simulink model "FSAC2021"  (R2014a)
settings: Solver=FixedStepDiscrete  StartTime=0.0  StopTime=inf  FixedStep=0.0005  RelTol=1e-3
model workspace (MAT data in the model file):
  MCOS : class17 (value not decoded)
  MCOS : class17 (value not decoded)
  MCOS : class17 (value not decoded)
  MCOS : class17 (value not decoded)
  MCOS : class17 (value not decoded)
  MCOS : class17 (value not decoded)
  MCOS : class17 (value not decoded)
  MCOS : class17 (value not decoded)
  MCOS : class17 (value not decoded)
  MCOS : class17 (value not decoded)
  MCOS : class17 (value not decoded)
  MCOS : class17 (value not decoded)
  MCOS : class17 (value not decoded)
  MCOS : class17 (value not decoded)
  MCOS : class17 (value not decoded)
  MCOS : class17 (value not decoded)
  MCOS : class17 (value not decoded)
  MCOS : class17 (value not decoded)
  MCOS : class17 (value not decoded)
  BUZZER_START = 1
  MCOS : class17 (value not decoded)
  MCOS : class17 (value not decoded)
  MCOS : class17 (value not decoded)
  MCOS : class17 (value not decoded)
  MCOS : class17 (value not decoded)
  MCOS : class17 (value not decoded)
  MCOS : class17 (value not decoded)
  MCOS : class17 (value not decoded)
  MCOS : class17 (value not decoded)
  MCOS : class17 (value not decoded)
  MCOS : class17 (value not decoded)
  MCOS : class17 (value not decoded)
  MCOS : class17 (value not decoded)
  MCOS : class17 (value not decoded)
  MCOS : class17 (value not decoded)
  MCOS : class17 (value not decoded)
  MCOS : class17 (value not decoded)
  MCOS : class17 (value not decoded)
  MCOS : class17 (value not decoded)
  MCOS : class17 (value not decoded)
  MCOS : class17 (value not decoded)
  MCOS : class17 (value not decoded)
  MCOS : class17 (value not decoded)
  MCOS : class17 (value not decoded)
  MCOS : class17 (value not decoded)
  MCOS : class17 (value not decoded)
  MCOS : class17 (value not decoded)
  MCOS : class17 (value not decoded)
  MCOS : class17 (value not decoded)
  MCOS : class17 (value not decoded)
  MCOS : class17 (value not decoded)
  MCOS : class17 (value not decoded)
  MCOS : class17 (value not decoded)
  MCOS : class17 (value not decoded)
  MCOS : class17 (value not decoded)
  MCOS : class17 (value not decoded)
  MCOS : class17 (value not decoded)
  MCOS : class17 (value not decoded)
  Brake = 11
  MCOS : class17 (value not decoded)
  MCOS : class17 (value not decoded)
  MCOS : class17 (value not decoded)
  MCOS : class17 (value not decoded)
  MCOS : class17 (value not decoded)
  MCOS : class17 (value not decoded)
  MCOS : class17 (value not decoded)
  MCOS : class17 (value not decoded)
  Sensor_Acc_b = 101.85
  Sensor_Acc_k = -0.0185
  Str_Sen_Orig_Angle = -341
  MCOS : class17 (value not decoded)
  Tire_D = 0.47
  T = 0.05
libraries: simulink x396, ec55xxlib x126
(part 10 of 17)

== system FSAC2021/ROUTING/TO_DCAN/Subsystem/DIAG_VEH_INFO ==
  Volt_Cmp_Mtr_Sts_in : Inport
  Volt_Cmp_BMS_Sts_in : Inport  Port=2
  Hydra_Prs_SN_Sts_in : Inport  Port=3
  EBS_Gas_SN_2_Sts_in : Inport  Port=4
  EBS_Gas_SN_1_Sts_in : Inport  Port=5
  Brk_Disp_SN_Sts_in : Inport  Port=6
  Acc_SN_2_Sts_in : Inport  Port=7
  Acc_SN_1_Sts_in : Inport  Port=8
  Point_VCU_in : Inport  Port=9
  Point_StrSr_in : Inport  Port=10
  Point_SCU_in : Inport  Port=11
  Point_RES_in : Inport  Port=12
  Point_MCU_in : Inport  Port=13
  Point_IPC_in : Inport  Port=14
  Point_Drive_Motor_in : Inport  Port=15
  Point_BMS_in : Inport  Port=16
  Point_BCU_in : Inport  Port=17
  Start_Swtich_in : Inport  Port=18
  On_Out_Switch_in : Inport  Port=19
  On_In_Swtich_in : Inport  Port=20
  LV_Switch_in : Inport  Port=21
  HV_Switch_in : Inport  Port=22
  EBS_Rls_Switch_in : Inport  Port=23
  ASMS_Swtich_in : Inport  Port=24
  AMI_State_in : Inport  Port=25
  High_voltage_on_in : Inport  Port=26
  EBS_Status_in : Inport  Port=27
  EBS_Fault_in : Inport  Port=28
  AS_State_in : Inport  Port=29
  AMI_State : Subsystem
  ASMS_Swtich : Subsystem
  AS_State : Subsystem
  Acc_SN_1_Sts : Subsystem
  Acc_SN_2_Sts : Subsystem
  Brk_Disp_SN_Sts : Subsystem
  Conv{1..8} (8 alike) : DataTypeConversion
  DIAG_VEH_INFO_DLC : Constant  Value=8  OutDataTypeStr=uint8
  DIAG_VEH_INFO_DLC_Out : Terminator
  DIAG_VEH_INFO_ID : Constant  Value=1905  OutDataTypeStr=single
  DIAG_VEH_INFO_ID_Out : Terminator
  DIAG_VEH_INFO_mux : Mux  Inputs=8
  EBS_Fault : Subsystem
  EBS_Gas_SN_1_Sts : Subsystem
  EBS_Gas_SN_2_Sts : Subsystem
  EBS_Rls_Switch : Subsystem
  EBS_Status : Subsystem
  HV_Switch : Subsystem
  High_voltage_on : Subsystem
  Hydra_Prs_SN_Sts : Subsystem
  LV_Switch : Subsystem
  On_In_Swtich : Subsystem
  On_Out_Switch : Subsystem
  Point_BCU : Subsystem
  Point_BMS : Subsystem
  Point_Drive_Motor : Subsystem
  Point_IPC : Subsystem
  Point_MCU : Subsystem
  Point_RES : Subsystem
  Point_SCU : Subsystem
  Point_StrSr : Subsystem
  Point_VCU : Subsystem
  Start_Swtich : Subsystem
  Volt_Cmp_BMS_Sts : Subsystem
  Volt_Cmp_Mtr_Sts : Subsystem
  or{1..8} (8 alike) : simulink/Logic and Bit Operations/Bitwise Operator  logicop=OR  UseBitMask=off  NumInputPorts=29  BitMask=bin2dec('11011001')  BitMaskRealWorld=Stored Integer
  output : Outport
  wires:
  DIAG_VEH_INFO_mux/1 -> output/1
  Volt_Cmp_Mtr_Sts/1(output1) -> or1/1
  Volt_Cmp_Mtr_Sts/2(output2) -> or2/1
  Volt_Cmp_Mtr_Sts/3(output3) -> or3/1
  Volt_Cmp_Mtr_Sts/4(output4) -> or4/1
  Volt_Cmp_Mtr_Sts/5(output5) -> or5/1
  Volt_Cmp_Mtr_Sts/6(output6) -> or6/1
  Volt_Cmp_Mtr_Sts/7(output7) -> or7/1
  Volt_Cmp_Mtr_Sts/8(output8) -> or8/1
  Volt_Cmp_BMS_Sts/1(output1) -> or1/2
  Volt_Cmp_BMS_Sts/2(output2) -> or2/2
  Volt_Cmp_BMS_Sts/3(output3) -> or3/2
  Volt_Cmp_BMS_Sts/4(output4) -> or4/2
  Volt_Cmp_BMS_Sts/5(output5) -> or5/2
  Volt_Cmp_BMS_Sts/6(output6) -> or6/2
  Volt_Cmp_BMS_Sts/7(output7) -> or7/2
  Volt_Cmp_BMS_Sts/8(output8) -> or8/2
  Hydra_Prs_SN_Sts/1(output1) -> or1/3
  Hydra_Prs_SN_Sts/2(output2) -> or2/3
  Hydra_Prs_SN_Sts/3(output3) -> or3/3
  Hydra_Prs_SN_Sts/4(output4) -> or4/3
  Hydra_Prs_SN_Sts/5(output5) -> or5/3
  Hydra_Prs_SN_Sts/6(output6) -> or6/3
  Hydra_Prs_SN_Sts/7(output7) -> or7/3
  Hydra_Prs_SN_Sts/8(output8) -> or8/3
  EBS_Gas_SN_2_Sts/1(output1) -> or1/4
  EBS_Gas_SN_2_Sts/2(output2) -> or2/4
  EBS_Gas_SN_2_Sts/3(output3) -> or3/4
  EBS_Gas_SN_2_Sts/4(output4) -> or4/4
  EBS_Gas_SN_2_Sts/5(output5) -> or5/4
  EBS_Gas_SN_2_Sts/6(output6) -> or6/4
  EBS_Gas_SN_2_Sts/7(output7) -> or7/4
  EBS_Gas_SN_2_Sts/8(output8) -> or8/4
  EBS_Gas_SN_1_Sts/1(output1) -> or1/5
  EBS_Gas_SN_1_Sts/2(output2) -> or2/5
  EBS_Gas_SN_1_Sts/3(output3) -> or3/5
  EBS_Gas_SN_1_Sts/4(output4) -> or4/5
  EBS_Gas_SN_1_Sts/5(output5) -> or5/5
  EBS_Gas_SN_1_Sts/6(output6) -> or6/5
  EBS_Gas_SN_1_Sts/7(output7) -> or7/5
  EBS_Gas_SN_1_Sts/8(output8) -> or8/5
  Brk_Disp_SN_Sts/1(output1) -> or1/6
  Brk_Disp_SN_Sts/2(output2) -> or2/6
  Brk_Disp_SN_Sts/3(output3) -> or3/6
  Brk_Disp_SN_Sts/4(output4) -> or4/6
  Brk_Disp_SN_Sts/5(output5) -> or5/6
  Brk_Disp_SN_Sts/6(output6) -> or6/6
  Brk_Disp_SN_Sts/7(output7) -> or7/6
  Brk_Disp_SN_Sts/8(output8) -> or8/6
  Acc_SN_2_Sts/1(output1) -> or1/7
  Acc_SN_2_Sts/2(output2) -> or2/7
  Acc_SN_2_Sts/3(output3) -> or3/7
  Acc_SN_2_Sts/4(output4) -> or4/7
  Acc_SN_2_Sts/5(output5) -> or5/7
  Acc_SN_2_Sts/6(output6) -> or6/7
  Acc_SN_2_Sts/7(output7) -> or7/7
  Acc_SN_2_Sts/8(output8) -> or8/7
  Acc_SN_1_Sts/1(output1) -> or1/8
  Acc_SN_1_Sts/2(output2) -> or2/8
  Acc_SN_1_Sts/3(output3) -> or3/8
  Acc_SN_1_Sts/4(output4) -> or4/8
  Acc_SN_1_Sts/5(output5) -> or5/8
  Acc_SN_1_Sts/6(output6) -> or6/8
  Acc_SN_1_Sts/7(output7) -> or7/8
  Acc_SN_1_Sts/8(output8) -> or8/8
  Point_VCU/1(output1) -> or1/9
  Point_VCU/2(output2) -> or2/9
  Point_VCU/3(output3) -> or3/9
  Point_VCU/4(output4) -> or4/9
  Point_VCU/5(output5) -> or5/9
  Point_VCU/6(output6) -> or6/9
  Point_VCU/7(output7) -> or7/9
  Point_VCU/8(output8) -> or8/9
  Point_StrSr/1(output1) -> or1/10
  Point_StrSr/2(output2) -> or2/10
  Point_StrSr/3(output3) -> or3/10
  Point_StrSr/4(output4) -> or4/10
  Point_StrSr/5(output5) -> or5/10
  Point_StrSr/6(output6) -> or6/10
  Point_StrSr/7(output7) -> or7/10
  Point_StrSr/8(output8) -> or8/10
  Point_SCU/1(output1) -> or1/11
  Point_SCU/2(output2) -> or2/11
  Point_SCU/3(output3) -> or3/11
  Point_SCU/4(output4) -> or4/11
  Point_SCU/5(output5) -> or5/11
  Point_SCU/6(output6) -> or6/11
  Point_SCU/7(output7) -> or7/11
  Point_SCU/8(output8) -> or8/11
  Point_RES/1(output1) -> or1/12
  Point_RES/2(output2) -> or2/12
  Point_RES/3(output3) -> or3/12
  Point_RES/4(output4) -> or4/12
  Point_RES/5(output5) -> or5/12
  Point_RES/6(output6) -> or6/12
  Point_RES/7(output7) -> or7/12
  Point_RES/8(output8) -> or8/12
  Point_MCU/1(output1) -> or1/13
  Point_MCU/2(output2) -> or2/13
  Point_MCU/3(output3) -> or3/13
  Point_MCU/4(output4) -> or4/13
  Point_MCU/5(output5) -> or5/13
  Point_MCU/6(output6) -> or6/13
  Point_MCU/7(output7) -> or7/13
  Point_MCU/8(output8) -> or8/13
  Point_IPC/1(output1) -> or1/14
  Point_IPC/2(output2) -> or2/14
  Point_IPC/3(output3) -> or3/14
  Point_IPC/4(output4) -> or4/14
  Point_IPC/5(output5) -> or5/14
  Point_IPC/6(output6) -> or6/14
  Point_IPC/7(output7) -> or7/14
  Point_IPC/8(output8) -> or8/14
  Point_Drive_Motor/1(output1) -> or1/15
  Point_Drive_Motor/2(output2) -> or2/15
  Point_Drive_Motor/3(output3) -> or3/15
  Point_Drive_Motor/4(output4) -> or4/15
  Point_Drive_Motor/5(output5) -> or5/15
  Point_Drive_Motor/6(output6) -> or6/15
  Point_Drive_Motor/7(output7) -> or7/15
  Point_Drive_Motor/8(output8) -> or8/15
  Point_BMS/1(output1) -> or1/16
  Point_BMS/2(output2) -> or2/16
  Point_BMS/3(output3) -> or3/16
  Point_BMS/4(output4) -> or4/16
  Point_BMS/5(output5) -> or5/16
  Point_BMS/6(output6) -> or6/16
  Point_BMS/7(output7) -> or7/16
  Point_BMS/8(output8) -> or8/16
  Point_BCU/1(output1) -> or1/17
  Point_BCU/2(output2) -> or2/17
  Point_BCU/3(output3) -> or3/17
  Point_BCU/4(output4) -> or4/17
  Point_BCU/5(output5) -> or5/17
  Point_BCU/6(output6) -> or6/17
  Point_BCU/7(output7) -> or7/17
  Point_BCU/8(output8) -> or8/17
  Start_Swtich/1(output1) -> or1/18
  Start_Swtich/2(output2) -> or2/18
  Start_Swtich/3(output3) -> or3/18
  Start_Swtich/4(output4) -> or4/18
  Start_Swtich/5(output5) -> or5/18
  Start_Swtich/6(output6) -> or6/18
  Start_Swtich/7(output7) -> or7/18
  Start_Swtich/8(output8) -> or8/18
  On_Out_Switch/1(output1) -> or1/19
  On_Out_Switch/2(output2) -> or2/19
  On_Out_Switch/3(output3) -> or3/19
  On_Out_Switch/4(output4) -> or4/19
  On_Out_Switch/5(output5) -> or5/19
  On_Out_Switch/6(output6) -> or6/19
  On_Out_Switch/7(output7) -> or7/19
  On_Out_Switch/8(output8) -> or8/19
  On_In_Swtich/1(output1) -> or1/20
  On_In_Swtich/2(output2) -> or2/20
  On_In_Swtich/3(output3) -> or3/20
  On_In_Swtich/4(output4) -> or4/20
  On_In_Swtich/5(output5) -> or5/20
  On_In_Swtich/6(output6) -> or6/20
  On_In_Swtich/7(output7) -> or7/20
  On_In_Swtich/8(output8) -> or8/20
  LV_Switch/1(output1) -> or1/21
  LV_Switch/2(output2) -> or2/21
  LV_Switch/3(output3) -> or3/21
  LV_Switch/4(output4) -> or4/21
  LV_Switch/5(output5) -> or5/21
  LV_Switch/6(output6) -> or6/21
  LV_Switch/7(output7) -> or7/21
  LV_Switch/8(output8) -> or8/21
  HV_Switch/1(output1) -> or1/22
  HV_Switch/2(output2) -> or2/22
  HV_Switch/3(output3) -> or3/22
  HV_Switch/4(output4) -> or4/22
  HV_Switch/5(output5) -> or5/22
  HV_Switch/6(output6) -> or6/22
  HV_Switch/7(output7) -> or7/22
  HV_Switch/8(output8) -> or8/22
  EBS_Rls_Switch/1(output1) -> or1/23
  EBS_Rls_Switch/2(output2) -> or2/23
  EBS_Rls_Switch/3(output3) -> or3/23
  EBS_Rls_Switch/4(output4) -> or4/23
  EBS_Rls_Switch/5(output5) -> or5/23
  EBS_Rls_Switch/6(output6) -> or6/23
  EBS_Rls_Switch/7(output7) -> or7/23
  EBS_Rls_Switch/8(output8) -> or8/23
  ASMS_Swtich/1(output1) -> or1/24
  ASMS_Swtich/2(output2) -> or2/24
  ASMS_Swtich/3(output3) -> or3/24
  ASMS_Swtich/4(output4) -> or4/24
  ASMS_Swtich/5(output5) -> or5/24
  ASMS_Swtich/6(output6) -> or6/24
  ASMS_Swtich/7(output7) -> or7/24
  ASMS_Swtich/8(output8) -> or8/24
  AMI_State/1(output1) -> or1/25
  AMI_State/2(output2) -> or2/25
  AMI_State/3(output3) -> or3/25
  AMI_State/4(output4) -> or4/25
  AMI_State/5(output5) -> or5/25
  AMI_State/6(output6) -> or6/25
  AMI_State/7(output7) -> or7/25
  AMI_State/8(output8) -> or8/25
  High_voltage_on/1(output1) -> or1/26
  High_voltage_on/2(output2) -> or2/26
  High_voltage_on/3(output3) -> or3/26
  High_voltage_on/4(output4) -> or4/26
  High_voltage_on/5(output5) -> or5/26
  High_voltage_on/6(output6) -> or6/26
  High_voltage_on/7(output7) -> or7/26
  High_voltage_on/8(output8) -> or8/26
  EBS_Status/1(output1) -> or1/27
  EBS_Status/2(output2) -> or2/27
  EBS_Status/3(output3) -> or3/27
  EBS_Status/4(output4) -> or4/27
  EBS_Status/5(output5) -> or5/27
  EBS_Status/6(output6) -> or6/27
  EBS_Status/7(output7) -> or7/27
  EBS_Status/8(output8) -> or8/27
  EBS_Fault/1(output1) -> or1/28
  EBS_Fault/2(output2) -> or2/28
  EBS_Fault/3(output3) -> or3/28
  EBS_Fault/4(output4) -> or4/28
  EBS_Fault/5(output5) -> or5/28
  EBS_Fault/6(output6) -> or6/28
  EBS_Fault/7(output7) -> or7/28
  EBS_Fault/8(output8) -> or8/28
  AS_State/1(output1) -> or1/29
  AS_State/2(output2) -> or2/29
  AS_State/3(output3) -> or3/29
  AS_State/4(output4) -> or4/29
  AS_State/5(output5) -> or5/29
  AS_State/6(output6) -> or6/29
  AS_State/7(output7) -> or7/29
  AS_State/8(output8) -> or8/29
  or1/1 -> Conv1/1
  Conv1/1 -> DIAG_VEH_INFO_mux/1
  or2/1 -> Conv2/1
  Conv2/1 -> DIAG_VEH_INFO_mux/2
  or3/1 -> Conv3/1
  Conv3/1 -> DIAG_VEH_INFO_mux/3
  or4/1 -> Conv4/1
  Conv4/1 -> DIAG_VEH_INFO_mux/4
  or5/1 -> Conv5/1
  Conv5/1 -> DIAG_VEH_INFO_mux/5
  or6/1 -> Conv6/1
  Conv6/1 -> DIAG_VEH_INFO_mux/6
  or7/1 -> Conv7/1
  Conv7/1 -> DIAG_VEH_INFO_mux/7
  or8/1 -> Conv8/1
  Conv8/1 -> DIAG_VEH_INFO_mux/8
  DIAG_VEH_INFO_ID/1 -> DIAG_VEH_INFO_ID_Out/1
  DIAG_VEH_INFO_DLC/1 -> DIAG_VEH_INFO_DLC_Out/1
  Volt_Cmp_Mtr_Sts_in/1 -> Volt_Cmp_Mtr_Sts/1(Volt_Cmp_Mtr_Sts)
  Volt_Cmp_BMS_Sts_in/1 -> Volt_Cmp_BMS_Sts/1(Volt_Cmp_BMS_Sts)
  Hydra_Prs_SN_Sts_in/1 -> Hydra_Prs_SN_Sts/1(Hydra_Prs_SN_Sts)
  EBS_Gas_SN_2_Sts_in/1 -> EBS_Gas_SN_2_Sts/1(EBS_Gas_SN_2_Sts)
  EBS_Gas_SN_1_Sts_in/1 -> EBS_Gas_SN_1_Sts/1(EBS_Gas_SN_1_Sts)
  Brk_Disp_SN_Sts_in/1 -> Brk_Disp_SN_Sts/1(Brk_Disp_SN_Sts)
  Acc_SN_2_Sts_in/1 -> Acc_SN_2_Sts/1(Acc_SN_2_Sts)
  Acc_SN_1_Sts_in/1 -> Acc_SN_1_Sts/1(Acc_SN_1_Sts)
  Point_VCU_in/1 -> Point_VCU/1(Point_VCU)
  Point_StrSr_in/1 -> Point_StrSr/1(Point_StrSr)
  Point_SCU_in/1 -> Point_SCU/1(Point_SCU)
  Point_RES_in/1 -> Point_RES/1(Point_RES)
  Point_MCU_in/1 -> Point_MCU/1(Point_MCU)
  Point_IPC_in/1 -> Point_IPC/1(Point_IPC)
  Point_Drive_Motor_in/1 -> Point_Drive_Motor/1(Point_Drive_Motor)
  Point_BMS_in/1 -> Point_BMS/1(Point_BMS)
  Point_BCU_in/1 -> Point_BCU/1(Point_BCU)
  Start_Swtich_in/1 -> Start_Swtich/1(Start_Swtich)
  On_Out_Switch_in/1 -> On_Out_Switch/1(On_Out_Switch)
  On_In_Swtich_in/1 -> On_In_Swtich/1(On_In_Swtich)
  LV_Switch_in/1 -> LV_Switch/1(LV_Switch)
  HV_Switch_in/1 -> HV_Switch/1(HV_Switch)
  EBS_Rls_Switch_in/1 -> EBS_Rls_Switch/1(EBS_Rls_Switch)
  ASMS_Swtich_in/1 -> ASMS_Swtich/1(ASMS_Swtich)
  AMI_State_in/1 -> AMI_State/1(AMI_State)
  High_voltage_on_in/1 -> High_voltage_on/1(High_voltage_on)
  EBS_Status_in/1 -> EBS_Status/1(EBS_Status)
  EBS_Fault_in/1 -> EBS_Fault/1(EBS_Fault)
  AS_State_in/1 -> AS_State/1(AS_State)

== system FSAC2021/ROUTING/TO_DCAN/Subsystem/DIAG_VEH_SENSOR ==
  Pedal_Brake_in : Inport
  Pedal_Acc_in : Inport  Port=2
  Veh_Current_Speed_in : Inport  Port=3
  Front_wheel_angle_in : Inport  Port=4
  Mtr_Input_Volt_in : Inport  Port=5
  BMS_Output_Volt_in : Inport  Port=6
  Hydra_Prs_in : Inport  Port=7
  EBS_Gas_Prs_2_in : Inport  Port=8
  EBS_Gas_Prs_1_in : Inport  Port=9
  BMS_Output_Volt : Subsystem
  Conv{1..8} (8 alike) : DataTypeConversion
  DIAG_VEH_SENSOR_DLC : Constant  Value=8  OutDataTypeStr=uint8
  DIAG_VEH_SENSOR_DLC_Out : Terminator
  DIAG_VEH_SENSOR_ID : Constant  Value=1873  OutDataTypeStr=single
  DIAG_VEH_SENSOR_ID_Out : Terminator
  DIAG_VEH_SENSOR_mux : Mux  Inputs=8
  EBS_Gas_Prs_1 : Subsystem
  EBS_Gas_Prs_2 : Subsystem
  Front_wheel_angle : Subsystem
  Hydra_Prs : Subsystem
  Mtr_Input_Volt : Subsystem
  Pedal_Acc : Subsystem
  Pedal_Brake : Subsystem
  Veh_Current_Speed : Subsystem
  or{1..8} (8 alike) : simulink/Logic and Bit Operations/Bitwise Operator  logicop=OR  UseBitMask=off  NumInputPorts=9  BitMask=bin2dec('11011001')  BitMaskRealWorld=Stored Integer
  output : Outport
  wires:
  DIAG_VEH_SENSOR_mux/1 -> output/1
  Pedal_Brake/1(output1) -> or1/1
  Pedal_Brake/2(output2) -> or2/1
  Pedal_Brake/3(output3) -> or3/1
  Pedal_Brake/4(output4) -> or4/1
  Pedal_Brake/5(output5) -> or5/1
  Pedal_Brake/6(output6) -> or6/1
  Pedal_Brake/7(output7) -> or7/1
  Pedal_Brake/8(output8) -> or8/1
  Pedal_Acc/1(output1) -> or1/2
  Pedal_Acc/2(output2) -> or2/2
  Pedal_Acc/3(output3) -> or3/2
  Pedal_Acc/4(output4) -> or4/2
  Pedal_Acc/5(output5) -> or5/2
  Pedal_Acc/6(output6) -> or6/2
  Pedal_Acc/7(output7) -> or7/2
  Pedal_Acc/8(output8) -> or8/2
  Veh_Current_Speed/1(output1) -> or1/3
  Veh_Current_Speed/2(output2) -> or2/3
  Veh_Current_Speed/3(output3) -> or3/3
  Veh_Current_Speed/4(output4) -> or4/3
  Veh_Current_Speed/5(output5) -> or5/3
  Veh_Current_Speed/6(output6) -> or6/3
  Veh_Current_Speed/7(output7) -> or7/3
  Veh_Current_Speed/8(output8) -> or8/3
  Front_wheel_angle/1(output1) -> or1/4
  Front_wheel_angle/2(output2) -> or2/4
  Front_wheel_angle/3(output3) -> or3/4
  Front_wheel_angle/4(output4) -> or4/4
  Front_wheel_angle/5(output5) -> or5/4
  Front_wheel_angle/6(output6) -> or6/4
  Front_wheel_angle/7(output7) -> or7/4
  Front_wheel_angle/8(output8) -> or8/4
  Mtr_Input_Volt/1(output1) -> or1/5
  Mtr_Input_Volt/2(output2) -> or2/5
  Mtr_Input_Volt/3(output3) -> or3/5
  Mtr_Input_Volt/4(output4) -> or4/5
  Mtr_Input_Volt/5(output5) -> or5/5
  Mtr_Input_Volt/6(output6) -> or6/5
  Mtr_Input_Volt/7(output7) -> or7/5
  Mtr_Input_Volt/8(output8) -> or8/5
  BMS_Output_Volt/1(output1) -> or1/6
  BMS_Output_Volt/2(output2) -> or2/6
  BMS_Output_Volt/3(output3) -> or3/6
  BMS_Output_Volt/4(output4) -> or4/6
  BMS_Output_Volt/5(output5) -> or5/6
  BMS_Output_Volt/6(output6) -> or6/6
  BMS_Output_Volt/7(output7) -> or7/6
  BMS_Output_Volt/8(output8) -> or8/6
  Hydra_Prs/1(output1) -> or1/7
  Hydra_Prs/2(output2) -> or2/7
  Hydra_Prs/3(output3) -> or3/7
  Hydra_Prs/4(output4) -> or4/7
  Hydra_Prs/5(output5) -> or5/7
  Hydra_Prs/6(output6) -> or6/7
  Hydra_Prs/7(output7) -> or7/7
  Hydra_Prs/8(output8) -> or8/7
  EBS_Gas_Prs_2/1(output1) -> or1/8
  EBS_Gas_Prs_2/2(output2) -> or2/8
  EBS_Gas_Prs_2/3(output3) -> or3/8
  EBS_Gas_Prs_2/4(output4) -> or4/8
  EBS_Gas_Prs_2/5(output5) -> or5/8
  EBS_Gas_Prs_2/6(output6) -> or6/8
  EBS_Gas_Prs_2/7(output7) -> or7/8
  EBS_Gas_Prs_2/8(output8) -> or8/8
  EBS_Gas_Prs_1/1(output1) -> or1/9
  EBS_Gas_Prs_1/2(output2) -> or2/9
  EBS_Gas_Prs_1/3(output3) -> or3/9
  EBS_Gas_Prs_1/4(output4) -> or4/9
  EBS_Gas_Prs_1/5(output5) -> or5/9
  EBS_Gas_Prs_1/6(output6) -> or6/9
  EBS_Gas_Prs_1/7(output7) -> or7/9
  EBS_Gas_Prs_1/8(output8) -> or8/9
  or1/1 -> Conv1/1
  Conv1/1 -> DIAG_VEH_SENSOR_mux/1
  or2/1 -> Conv2/1
  Conv2/1 -> DIAG_VEH_SENSOR_mux/2
  or3/1 -> Conv3/1
  Conv3/1 -> DIAG_VEH_SENSOR_mux/3
  or4/1 -> Conv4/1
  Conv4/1 -> DIAG_VEH_SENSOR_mux/4
  or5/1 -> Conv5/1
  Conv5/1 -> DIAG_VEH_SENSOR_mux/5
  or6/1 -> Conv6/1
  Conv6/1 -> DIAG_VEH_SENSOR_mux/6
  or7/1 -> Conv7/1
  Conv7/1 -> DIAG_VEH_SENSOR_mux/7
  or8/1 -> Conv8/1
  Conv8/1 -> DIAG_VEH_SENSOR_mux/8
  DIAG_VEH_SENSOR_ID/1 -> DIAG_VEH_SENSOR_ID_Out/1
  DIAG_VEH_SENSOR_DLC/1 -> DIAG_VEH_SENSOR_DLC_Out/1
  Pedal_Brake_in/1 -> Pedal_Brake/1(Pedal_Brake)
  Pedal_Acc_in/1 -> Pedal_Acc/1(Pedal_Acc)
  Veh_Current_Speed_in/1 -> Veh_Current_Speed/1(Veh_Current_Speed)
  Front_wheel_angle_in/1 -> Front_wheel_angle/1(Front_wheel_angle)
  Mtr_Input_Volt_in/1 -> Mtr_Input_Volt/1(Mtr_Input_Volt)
  BMS_Output_Volt_in/1 -> BMS_Output_Volt/1(BMS_Output_Volt)
  Hydra_Prs_in/1 -> Hydra_Prs/1(Hydra_Prs)
  EBS_Gas_Prs_2_in/1 -> EBS_Gas_Prs_2/1(EBS_Gas_Prs_2)
  EBS_Gas_Prs_1_in/1 -> EBS_Gas_Prs_1/1(EBS_Gas_Prs_1)

== system FSAC2021/ROUTING/TO_DCAN/Subsystem/DIAG_WHL_SPD ==
  RR_Whl_Spd_in : Inport
  FR_Whl_Spd_in : Inport  Port=2
  RL_Whl_Spd_in : Inport  Port=3
  FL_Whl_Spd_in : Inport  Port=4
  Conv{1..8} (8 alike) : DataTypeConversion
  DIAG_WHL_SPD_DLC : Constant  Value=8  OutDataTypeStr=uint8
  DIAG_WHL_SPD_DLC_Out : Terminator
  DIAG_WHL_SPD_ID : Constant  Value=1889  OutDataTypeStr=single
  DIAG_WHL_SPD_ID_Out : Terminator
  DIAG_WHL_SPD_mux : Mux  Inputs=8
  FL_Whl_Spd : Subsystem
  FR_Whl_Spd : Subsystem
  RL_Whl_Spd : Subsystem
  RR_Whl_Spd : Subsystem
  or{1..8} (8 alike) : simulink/Logic and Bit Operations/Bitwise Operator  logicop=OR  UseBitMask=off  NumInputPorts=4  BitMask=bin2dec('11011001')  BitMaskRealWorld=Stored Integer
  output : Outport
  wires:
  DIAG_WHL_SPD_mux/1 -> output/1
  RR_Whl_Spd/1(output1) -> or1/1
  RR_Whl_Spd/2(output2) -> or2/1
  RR_Whl_Spd/3(output3) -> or3/1
  RR_Whl_Spd/4(output4) -> or4/1
  RR_Whl_Spd/5(output5) -> or5/1
  RR_Whl_Spd/6(output6) -> or6/1
  RR_Whl_Spd/7(output7) -> or7/1
  RR_Whl_Spd/8(output8) -> or8/1
  FR_Whl_Spd/1(output1) -> or1/2
  FR_Whl_Spd/2(output2) -> or2/2
  FR_Whl_Spd/3(output3) -> or3/2
  FR_Whl_Spd/4(output4) -> or4/2
  FR_Whl_Spd/5(output5) -> or5/2
  FR_Whl_Spd/6(output6) -> or6/2
  FR_Whl_Spd/7(output7) -> or7/2
  FR_Whl_Spd/8(output8) -> or8/2
  RL_Whl_Spd/1(output1) -> or1/3
  RL_Whl_Spd/2(output2) -> or2/3
  RL_Whl_Spd/3(output3) -> or3/3
  RL_Whl_Spd/4(output4) -> or4/3
  RL_Whl_Spd/5(output5) -> or5/3
  RL_Whl_Spd/6(output6) -> or6/3
  RL_Whl_Spd/7(output7) -> or7/3
  RL_Whl_Spd/8(output8) -> or8/3
  FL_Whl_Spd/1(output1) -> or1/4
  FL_Whl_Spd/2(output2) -> or2/4
  FL_Whl_Spd/3(output3) -> or3/4
  FL_Whl_Spd/4(output4) -> or4/4
  FL_Whl_Spd/5(output5) -> or5/4
  FL_Whl_Spd/6(output6) -> or6/4
  FL_Whl_Spd/7(output7) -> or7/4
  FL_Whl_Spd/8(output8) -> or8/4
  or1/1 -> Conv1/1
  Conv1/1 -> DIAG_WHL_SPD_mux/1
  or2/1 -> Conv2/1
  Conv2/1 -> DIAG_WHL_SPD_mux/2
  or3/1 -> Conv3/1
  Conv3/1 -> DIAG_WHL_SPD_mux/3
  or4/1 -> Conv4/1
  Conv4/1 -> DIAG_WHL_SPD_mux/4
  or5/1 -> Conv5/1
  Conv5/1 -> DIAG_WHL_SPD_mux/5
  or6/1 -> Conv6/1
  Conv6/1 -> DIAG_WHL_SPD_mux/6
  or7/1 -> Conv7/1
  Conv7/1 -> DIAG_WHL_SPD_mux/7
  or8/1 -> Conv8/1
  Conv8/1 -> DIAG_WHL_SPD_mux/8
  DIAG_WHL_SPD_ID/1 -> DIAG_WHL_SPD_ID_Out/1
  DIAG_WHL_SPD_DLC/1 -> DIAG_WHL_SPD_DLC_Out/1
  RR_Whl_Spd_in/1 -> RR_Whl_Spd/1(RR_Whl_Spd)
  FR_Whl_Spd_in/1 -> FR_Whl_Spd/1(FR_Whl_Spd)
  RL_Whl_Spd_in/1 -> RL_Whl_Spd/1(RL_Whl_Spd)
  FL_Whl_Spd_in/1 -> FL_Whl_Spd/1(FL_Whl_Spd)

== system FSAC2021/VCU_CAN_Read/DCAN_REC/DIAG_VCU_CTRL1/TEST_Acc_Sub ==
  In1 : Inport
  Out1 : Outport
  wires:
  In1/1 -> Out1/1

== system FSAC2021/VCU_CAN_Read/DCAN_REC/DIAG_VCU_CTRL1/TEST_Brake_Sub ==
  In1 : Inport
  Out1 : Outport
  wires:
  In1/1 -> Out1/1

== system FSAC2021/VCU_CAN_Read/DCAN_REC/DIAG_VCU_CTRL1/TEST_EBS_Sub ==
  In1 : Inport
  Out1 : Outport
  wires:
  In1/1 -> Out1/1

== system FSAC2021/VCU_CAN_Read/DCAN_REC/DIAG_VCU_CTRL1/TEST_Go_Sub ==
  In1 : Inport
  Out1 : Outport
  wires:
  In1/1 -> Out1/1

== system FSAC2021/VCU_CAN_Read/DCAN_REC/DIAG_VCU_CTRL1/TEST_Steer_Sub ==
  In1 : Inport
  Out1 : Outport
  wires:
  In1/1 -> Out1/1

== system FSAC2021/VCU_CAN_Read/DCAN_REC/DIAG_VCU_CTRL1/Vel_Ctrl_Req_Sub ==
  In1 : Inport
  Out1 : Outport
  wires:
  In1/1 -> Out1/1

== system FSAC2021/VCU_CAN_Read/PCANA(RES、AMI、MOTEC、BRAKE、STEER_SENSOR、IPC)/AMI_DUTY/assi_status_Sub ==
  In1 : Inport
  Out1 : Outport
  wires:
  In1/1 -> Out1/1

== system FSAC2021/VCU_CAN_Read/PCANA(RES、AMI、MOTEC、BRAKE、STEER_SENSOR、IPC)/BCU_MTR_STATUS1/Brake_cmd_fault_flag_Sub ==
  In1 : Inport
  Out1 : Outport
  wires:
  In1/1 -> Out1/1

== system FSAC2021/VCU_CAN_Read/PCANA(RES、AMI、MOTEC、BRAKE、STEER_SENSOR、IPC)/BCU_MTR_STATUS1/Brake_encoder_fault_sts_Sub ==
  In1 : Inport
  Out1 : Outport
  wires:
  In1/1 -> Out1/1

== system FSAC2021/VCU_CAN_Read/PCANA(RES、AMI、MOTEC、BRAKE、STEER_SENSOR、IPC)/BCU_MTR_STATUS1/Brake_go_origin_over_flag_Sub ==
  In1 : Inport
  Out1 : Outport
  wires:
  In1/1 -> Out1/1

== system FSAC2021/VCU_CAN_Read/PCANA(RES、AMI、MOTEC、BRAKE、STEER_SENSOR、IPC)/BCU_MTR_STATUS1/Brake_hd_fault_sts_Sub ==
  In1 : Inport
  Out1 : Outport
  wires:
  In1/1 -> Out1/1

== system FSAC2021/VCU_CAN_Read/PCANA(RES、AMI、MOTEC、BRAKE、STEER_SENSOR、IPC)/BCU_MTR_STATUS1/Brake_lowvolt_prtct_sts_Sub ==
  In1 : Inport
  Out1 : Outport
  wires:
  In1/1 -> Out1/1

== system FSAC2021/VCU_CAN_Read/PCANA(RES、AMI、MOTEC、BRAKE、STEER_SENSOR、IPC)/BCU_MTR_STATUS1/Brake_mtr_enable_flag_Sub ==
  In1 : Inport
  Out1 : Outport
  wires:
  In1/1 -> Out1/1

== system FSAC2021/VCU_CAN_Read/PCANA(RES、AMI、MOTEC、BRAKE、STEER_SENSOR、IPC)/BCU_MTR_STATUS1/Brake_mtr_goalpos_Sub ==
  In1 : Inport
  Out1 : Outport
  wires:
  In1/1 -> Out1/1

== system FSAC2021/VCU_CAN_Read/PCANA(RES、AMI、MOTEC、BRAKE、STEER_SENSOR、IPC)/BCU_MTR_STATUS1/Brake_mtr_origin_flag_Sub ==
  In1 : Inport
  Out1 : Outport
  wires:
  In1/1 -> Out1/1

== system FSAC2021/VCU_CAN_Read/PCANA(RES、AMI、MOTEC、BRAKE、STEER_SENSOR、IPC)/BCU_MTR_STATUS1/Brake_mtr_stop_flag_Sub ==
  In1 : Inport
  Out1 : Outport
  wires:
  In1/1 -> Out1/1

== system FSAC2021/VCU_CAN_Read/PCANA(RES、AMI、MOTEC、BRAKE、STEER_SENSOR、IPC)/BCU_MTR_STATUS1/Brake_offline_run_flag_Sub ==
  In1 : Inport
  Out1 : Outport
  wires:
  In1/1 -> Out1/1

== system FSAC2021/VCU_CAN_Read/PCANA(RES、AMI、MOTEC、BRAKE、STEER_SENSOR、IPC)/BCU_MTR_STATUS1/Brake_overcurrt_prtct_sts_Sub ==
  In1 : Inport
  Out1 : Outport
  wires:
  In1/1 -> Out1/1

== system FSAC2021/VCU_CAN_Read/PCANA(RES、AMI、MOTEC、BRAKE、STEER_SENSOR、IPC)/BCU_MTR_STATUS1/Brake_overheat_prtct_sts_Sub ==
  In1 : Inport
  Out1 : Outport
  wires:
  In1/1 -> Out1/1

== system FSAC2021/VCU_CAN_Read/PCANA(RES、AMI、MOTEC、BRAKE、STEER_SENSOR、IPC)/BCU_MTR_STATUS1/Brake_pos_enqual_Sub ==
  In1 : Inport
  Out1 : Outport
  wires:
  In1/1 -> Out1/1

== system FSAC2021/VCU_CAN_Read/PCANA(RES、AMI、MOTEC、BRAKE、STEER_SENSOR、IPC)/BCU_MTR_STATUS1/Brake_reg_rw_fault_flag_Sub ==
  In1 : Inport
  Out1 : Outport
  wires:
  In1/1 -> Out1/1

== system FSAC2021/VCU_CAN_Read/PCANA(RES、AMI、MOTEC、BRAKE、STEER_SENSOR、IPC)/BCU_MTR_STATUS1/Brake_sensor1_sts_Sub ==
  In1 : Inport
  Out1 : Outport
  wires:
  In1/1 -> Out1/1

== system FSAC2021/VCU_CAN_Read/PCANA(RES、AMI、MOTEC、BRAKE、STEER_SENSOR、IPC)/BCU_MTR_STATUS1/Brake_sensor2_sts_Sub ==
  In1 : Inport
  Out1 : Outport
  wires:
  In1/1 -> Out1/1

== system FSAC2021/VCU_CAN_Read/PCANA(RES、AMI、MOTEC、BRAKE、STEER_SENSOR、IPC)/BCU_MTR_STATUS1/Brake_sensor3_sts_Sub ==
  In1 : Inport
  Out1 : Outport
  wires:
  In1/1 -> Out1/1

== system FSAC2021/VCU_CAN_Read/PCANA(RES、AMI、MOTEC、BRAKE、STEER_SENSOR、IPC)/BCU_MTR_STATUS1/Brake_sensor4_sts_Sub ==
  In1 : Inport
  Out1 : Outport
  wires:
  In1/1 -> Out1/1

== system FSAC2021/VCU_CAN_Read/PCANA(RES、AMI、MOTEC、BRAKE、STEER_SENSOR、IPC)/BCU_MTR_STATUS1/Brake_sensor5_sts_Sub ==
  In1 : Inport
  Out1 : Outport
  wires:
  In1/1 -> Out1/1

== system FSAC2021/VCU_CAN_Read/PCANA(RES、AMI、MOTEC、BRAKE、STEER_SENSOR、IPC)/BCU_MTR_STATUS1/Brake_sensor6_sts_Sub ==
  In1 : Inport
  Out1 : Outport
  wires:
  In1/1 -> Out1/1

== system FSAC2021/VCU_CAN_Read/PCANA(RES、AMI、MOTEC、BRAKE、STEER_SENSOR、IPC)/BCU_MTR_STATUS1/Brake_speed_enqual_Sub ==
  In1 : Inport
  Out1 : Outport
  wires:
  In1/1 -> Out1/1

== system FSAC2021/VCU_CAN_Read/PCANA(RES、AMI、MOTEC、BRAKE、STEER_SENSOR、IPC)/Heartt/assi_status_Sub ==
  In1 : Inport
  Out1 : Outport
  wires:
  In1/1 -> Out1/1

== system FSAC2021/VCU_CAN_Read/PCANA(RES、AMI、MOTEC、BRAKE、STEER_SENSOR、IPC)/IPC_CMD1/IPC_Acc_Sub ==
  In1 : Inport
  Out1 : Outport
  wires:
  In1/1 -> Out1/1

== system FSAC2021/VCU_CAN_Read/PCANA(RES、AMI、MOTEC、BRAKE、STEER_SENSOR、IPC)/IPC_CMD1/IPC_Brk_Sub ==
  In1 : Inport
  Out1 : Outport
  wires:
  In1/1 -> Out1/1

== system FSAC2021/VCU_CAN_Read/PCANA(RES、AMI、MOTEC、BRAKE、STEER_SENSOR、IPC)/IPC_CMD1/IPC_Steer_Sub ==
  In1 : Inport
  Out1 : Outport
  wires:
  In1/1 -> Out1/1

== system FSAC2021/VCU_CAN_Read/PCANA(RES、AMI、MOTEC、BRAKE、STEER_SENSOR、IPC)/MOTEC_MOTION /MOTEC_MOTION ==
  input : Inport
  Demux : Demux  Outputs=8
  Motec_Currt_AngCS : ArithShift  BitShiftNumber=-16
  Motec_Currt_AngCS1 : ArithShift  BitShiftNumber=-15
  Motec_Currt_AngConS : Constant  OutDataTypeStr=single
  Motec_Currt_AngMinus : UnaryMinus
  Motec_Currt_AngROP : RelationalOperator  OutDataTypeStr=boolean
  Motec_Currt_AngSW : Switch  Criteria=u2 ~= 0
  Motec_Currt_Ang_Ad : Sum
  Motec_Currt_Ang_Convert : DataTypeConversion  OutDataTypeStr=uint32
  Motec_Currt_Ang_F : Gain  Gain=6
  Motec_Currt_Ang_L : simulink/Logic and Bit Operations/Bitwise Operator  logicop=AND  UseBitMask=on  BitMask=65535  BitMaskRealWorld=Stored Integer
  Motec_Currt_Ang_O : Constant  Value=0  OutDataTypeStr=single
  Motec_Currt_Ang_S : ArithShift
  Motec_Currt_Ang_Sub : Subsystem
  Motec_Currt_Ang_sat : Saturate  UpperLimit=196602  LowerLimit=-196608
  Motec_Currt_Angcv : DataTypeConversion
  Motec_Currt_Anginput6_Ad : Sum
  Motec_Currt_Anginput6_C : Constant  Value=256
  Motec_Currt_Anginput6_P : Product
  Motec_Currt_Angsubcon : Sum  Inputs=+-
  Motec_Currt_CurrentCS : ArithShift  BitShiftNumber=-16
  Motec_Currt_CurrentCS1 : ArithShift  BitShiftNumber=-15
  Motec_Currt_CurrentConS : Constant  OutDataTypeStr=single
  Motec_Currt_CurrentMinus : UnaryMinus
  Motec_Currt_CurrentROP : RelationalOperator  OutDataTypeStr=boolean
  Motec_Currt_CurrentSW : Switch  Criteria=u2 ~= 0
  Motec_Currt_Current_Ad : Sum
  Motec_Currt_Current_Convert : DataTypeConversion  OutDataTypeStr=uint32
  Motec_Currt_Current_F : Gain  Gain=0.001
  Motec_Currt_Current_L : simulink/Logic and Bit Operations/Bitwise Operator  logicop=AND  UseBitMask=on  BitMask=65535  BitMaskRealWorld=Stored Integer
  Motec_Currt_Current_O : Constant  Value=0  OutDataTypeStr=single
  Motec_Currt_Current_S : ArithShift
  Motec_Currt_Current_Sub : Subsystem
  Motec_Currt_Current_sat : Saturate  UpperLimit=32.767  LowerLimit=-32.768
  Motec_Currt_Currentcv : DataTypeConversion
  Motec_Currt_Currentinput8_Ad : Sum
  Motec_Currt_Currentinput8_C : Constant  Value=256
  Motec_Currt_Currentinput8_P : Product
  Motec_Currt_Currentsubcon : Sum  Inputs=+-
  Motec_Currt_PositionCMC : Constant  Value=0
  Motec_Currt_PositionCS : ArithShift  BitShiftNumber=-32
  Motec_Currt_PositionCS1 : ArithShift  BitShiftNumber=-31
  Motec_Currt_PositionConS : Constant  OutDataTypeStr=single
  Motec_Currt_PositionLOPCom : Logic  Operator=OR  AllPortsSameDT=off  OutDataTypeStr=boolean
  Motec_Currt_PositionMinus : UnaryMinus
  Motec_Currt_PositionROP : RelationalOperator  Operator=>  OutDataTypeStr=boolean
  Motec_Currt_PositionROP1 : RelationalOperator  Operator===  OutDataTypeStr=boolean
  Motec_Currt_PositionROP3 : RelationalOperator  Operator===  OutDataTypeStr=boolean
  Motec_Currt_PositionSW : Switch  Criteria=u2 ~= 0
  Motec_Currt_Position_Ad : Sum
  Motec_Currt_Position_Convert : DataTypeConversion  OutDataTypeStr=uint32
  Motec_Currt_Position_F : Gain  Gain=0.00146
  Motec_Currt_Position_L : simulink/Logic and Bit Operations/Bitwise Operator  logicop=AND  UseBitMask=on  BitMask=4294967295  BitMaskRealWorld=Stored Integer
  Motec_Currt_Position_LOPCom1 : Logic  AllPortsSameDT=off  OutDataTypeStr=boolean
  Motec_Currt_Position_O : Constant  Value=0  OutDataTypeStr=single
  Motec_Currt_Position_S : ArithShift
  Motec_Currt_Position_Sub : Subsystem
  Motec_Currt_Position_sat : Saturate  UpperLimit=3135326.12462  LowerLimit=-3135326.12608
  Motec_Currt_Positioncv : DataTypeConversion
  Motec_Currt_Positioninput2_Ad : Sum
  Motec_Currt_Positioninput2_C : Constant  Value=256
  Motec_Currt_Positioninput2_P : Product
  Motec_Currt_Positioninput3_Ad : Sum
  Motec_Currt_Positioninput3_C : Constant  Value=65536
  Motec_Currt_Positioninput3_P : Product
  Motec_Currt_Positioninput4_Ad : Sum
  Motec_Currt_Positioninput4_C : Constant  Value=16777216
  Motec_Currt_Positioninput4_P : Product
  Motec_Currt_Positionsubcon : Sum  Inputs=+-
  Motec_Currt_Ang_Out : Outport
  Motec_Currt_Current_Out : Outport  Port=2
  Motec_Currt_Position_Out : Outport  Port=3
  wires:
  Motec_Currt_Ang_F/1 -> Motec_Currt_Ang_Ad/1
  Motec_Currt_Ang_O/1 -> Motec_Currt_Ang_Ad/2
  Motec_Currt_Ang_Ad/1 -> Motec_Currt_Ang_sat/1
  Motec_Currt_Ang_sat/1 -> Motec_Currt_Ang_Out/1
  Demux/6 -> Motec_Currt_Anginput6_P/1
  Motec_Currt_Anginput6_C/1 -> Motec_Currt_Anginput6_P/2
  Motec_Currt_Anginput6_P/1 -> Motec_Currt_Anginput6_Ad/1
  Demux/5 -> Motec_Currt_Anginput6_Ad/2
  Motec_Currt_Anginput6_Ad/1 -> Motec_Currt_Ang_Sub/1(In1)
  Motec_Currt_Ang_Sub/1(Out1) -> Motec_Currt_Ang_Convert/1
  Motec_Currt_Ang_Convert/1 -> Motec_Currt_Ang_L/1
  Motec_Currt_Ang_L/1 -> Motec_Currt_Ang_S/1
  Motec_Currt_Ang_S/1 -> Motec_Currt_Angcv/1
  Motec_Currt_Angcv/1 -> Motec_Currt_AngROP/1, Motec_Currt_Angsubcon/2, Motec_Currt_AngSW/3
  Motec_Currt_AngConS/1 -> Motec_Currt_AngCS/1, Motec_Currt_AngCS1/1
  Motec_Currt_AngCS1/1 -> Motec_Currt_AngROP/2
  Motec_Currt_AngCS/1 -> Motec_Currt_Angsubcon/1
  Motec_Currt_Angsubcon/1 -> Motec_Currt_AngMinus/1
  Motec_Currt_AngMinus/1 -> Motec_Currt_AngSW/1
  Motec_Currt_AngSW/1 -> Motec_Currt_Ang_F/1
  Motec_Currt_AngROP/1 -> Motec_Currt_AngSW/2
  Motec_Currt_Current_F/1 -> Motec_Currt_Current_Ad/1
  Motec_Currt_Current_O/1 -> Motec_Currt_Current_Ad/2
  Motec_Currt_Current_Ad/1 -> Motec_Currt_Current_sat/1
  Motec_Currt_Current_sat/1 -> Motec_Currt_Current_Out/1
  Demux/8 -> Motec_Currt_Currentinput8_P/1
  Motec_Currt_Currentinput8_C/1 -> Motec_Currt_Currentinput8_P/2
  Motec_Currt_Currentinput8_P/1 -> Motec_Currt_Currentinput8_Ad/1
  Demux/7 -> Motec_Currt_Currentinput8_Ad/2
  Motec_Currt_Currentinput8_Ad/1 -> Motec_Currt_Current_Sub/1(In1)
  Motec_Currt_Current_Sub/1(Out1) -> Motec_Currt_Current_Convert/1
  Motec_Currt_Current_Convert/1 -> Motec_Currt_Current_L/1
  Motec_Currt_Current_L/1 -> Motec_Currt_Current_S/1
  Motec_Currt_Current_S/1 -> Motec_Currt_Currentcv/1
  Motec_Currt_Currentcv/1 -> Motec_Currt_Currentsubcon/2, Motec_Currt_CurrentSW/3, Motec_Currt_CurrentROP/1
  Motec_Currt_CurrentConS/1 -> Motec_Currt_CurrentCS/1, Motec_Currt_CurrentCS1/1
  Motec_Currt_CurrentCS1/1 -> Motec_Currt_CurrentROP/2
  Motec_Currt_CurrentCS/1 -> Motec_Currt_Currentsubcon/1
  Motec_Currt_Currentsubcon/1 -> Motec_Currt_CurrentMinus/1
  Motec_Currt_CurrentMinus/1 -> Motec_Currt_CurrentSW/1
  Motec_Currt_CurrentSW/1 -> Motec_Currt_Current_F/1
  Motec_Currt_CurrentROP/1 -> Motec_Currt_CurrentSW/2
  Motec_Currt_Position_F/1 -> Motec_Currt_Position_Ad/1
  Motec_Currt_Position_O/1 -> Motec_Currt_Position_Ad/2
  Motec_Currt_Position_Ad/1 -> Motec_Currt_Position_sat/1
  Motec_Currt_Position_sat/1 -> Motec_Currt_Position_Out/1
  Demux/2 -> Motec_Currt_Positioninput2_P/1
  Motec_Currt_Positioninput2_C/1 -> Motec_Currt_Positioninput2_P/2
  Motec_Currt_Positioninput2_P/1 -> Motec_Currt_Positioninput2_Ad/1
  Demux/1 -> Motec_Currt_Positioninput2_Ad/2
  Demux/3 -> Motec_Currt_Positioninput3_P/1, Motec_Currt_PositionROP1/1
  Motec_Currt_Positioninput3_C/1 -> Motec_Currt_Positioninput3_P/2
  Motec_Currt_Positioninput3_P/1 -> Motec_Currt_Positioninput3_Ad/1
  Motec_Currt_Positioninput2_Ad/1 -> Motec_Currt_Positioninput3_Ad/2
  Demux/4 -> Motec_Currt_Positioninput4_P/1
  Motec_Currt_Positioninput4_C/1 -> Motec_Currt_Positioninput4_P/2
  Motec_Currt_Positioninput4_P/1 -> Motec_Currt_Positioninput4_Ad/1
  Motec_Currt_Positioninput3_Ad/1 -> Motec_Currt_Positioninput4_Ad/2
  Motec_Currt_Positioninput4_Ad/1 -> Motec_Currt_Position_Sub/1(In1)
  Motec_Currt_Position_Sub/1(Out1) -> Motec_Currt_Position_Convert/1
  Motec_Currt_Position_Convert/1 -> Motec_Currt_Position_L/1
  Motec_Currt_Position_L/1 -> Motec_Currt_Position_S/1
  Motec_Currt_Position_S/1 -> Motec_Currt_Positioncv/1
  Motec_Currt_Positioncv/1 -> Motec_Currt_PositionROP/1, Motec_Currt_Positionsubcon/2, Motec_Currt_PositionSW/3, Motec_Currt_PositionROP3/1
  Motec_Currt_PositionConS/1 -> Motec_Currt_PositionCS/1, Motec_Currt_PositionCS1/1
  Motec_Currt_PositionCS1/1 -> Motec_Currt_PositionROP/2, Motec_Currt_PositionROP3/2
  Motec_Currt_PositionCS/1 -> Motec_Currt_Positionsubcon/1
  Motec_Currt_Positionsubcon/1 -> Motec_Currt_PositionMinus/1
  Motec_Currt_PositionMinus/1 -> Motec_Currt_PositionSW/1
  Motec_Currt_PositionSW/1 -> Motec_Currt_Position_F/1
  Motec_Currt_PositionROP1/1 -> Motec_Currt_Position_LOPCom1/1
  Motec_Currt_PositionROP3/1 -> Motec_Currt_Position_LOPCom1/2
  Motec_Currt_Position_LOPCom1/1 -> Motec_Currt_PositionLOPCom/2
  Motec_Currt_PositionROP/1 -> Motec_Currt_PositionLOPCom/1
  Motec_Currt_PositionLOPCom/1 -> Motec_Currt_PositionSW/2
  Motec_Currt_PositionCMC/1 -> Motec_Currt_PositionROP1/2
  input/1 -> Demux/1

== system FSAC2021/VCU_CAN_Read/PCANA(RES、AMI、MOTEC、BRAKE、STEER_SENSOR、IPC)/STEER_SENSOR_INFO1/Str_Sensor_Curr_Angle_Sub ==
  In1 : Inport
  Out1 : Outport
  wires:
  In1/1 -> Out1/1
